simulink model "example_roboracer"  (R2024b)
settings: Solver=VariableStepAuto  StartTime=0.0  StopTime=inf  RelTol=1e-3
undefined symbols (not defined in the file or in its folder): gray
settings Model: Creator=tsamak  LastModifiedBy=tsamak
settings OptimizationCC: ZeroExternalMemoryAtStartup=off  ZeroInternalMemoryAtStartup=off  InitFltsAndDblsToZero=on
settings DebuggingCC: UnderSpecifiedDimensionMsg=warning
settings HardwareCC: ProdLongLongMode=on  TargetLongLongMode=on
settings SFSimCC: SimTargetLang=C++  GPUAcceleration=on  SimDLTargetLibrary=cudnn
settings RTWCC: TargetLang=C++  GenerateGPUCode=CUDA  GPUComputeCapability=3.5
settings GRTTargetCC: TargetLangStandard=C++11 (ISO)  CodeInterfacePackaging=C++ class

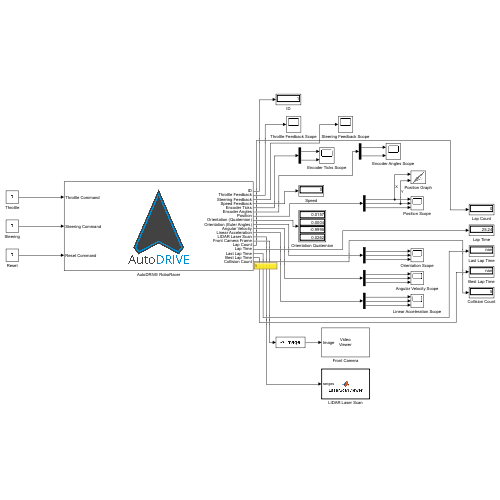
[thumbnail: Simulink's stored preview of the top-level diagram]
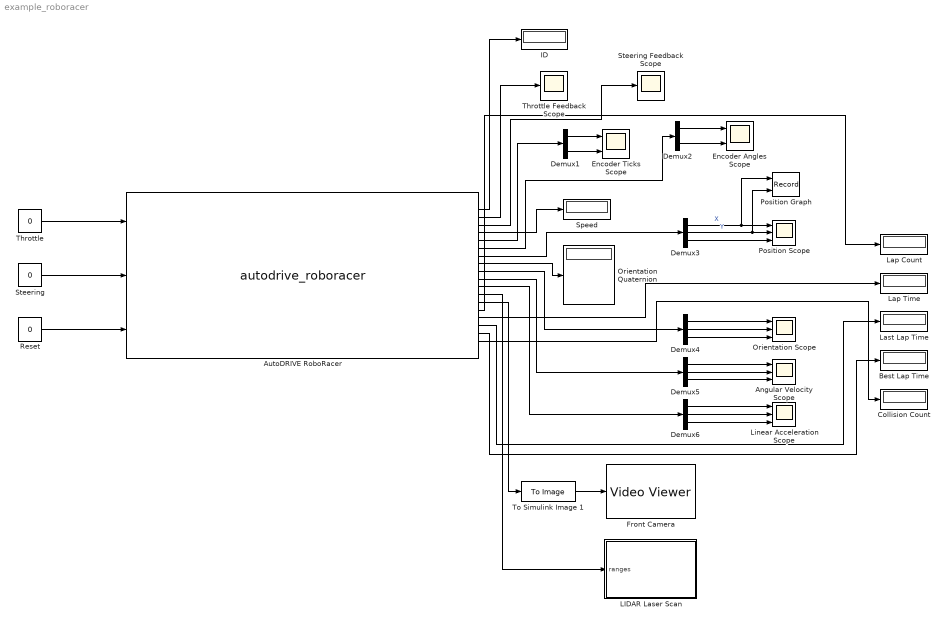
== system example_roboracer ==
  Angular Velocity Scope : Scope  NumInputPorts=3
  AutoDRIVE RoboRacer : M-S-Function  FunctionName=autodrive_roboracer  Parameters=Port  mask{Port=4567}
      mask Display:
      | image('autodrive_logo.png');
      | port_label('input', 1, 'Throttle Command');
      | port_label('input', 2, 'Steering Command');
      | port_label('input', 3, 'Reset Command');
      | port_label('output', 1, 'ID');
      | port_label('output', 2, 'Throttle Feedback');
      | port_label('output', 3, 'Steering Feedback');
      | port_label('output', 4, 'Speed Feedback');
      | port_label('output', 5, 'Encoder Ticks');
      | port_label('output', 6, 'Encoder Angles');
      | port_label('output', 7, 'Position');
      | port_label('output', 8, 'Orientation (Quaternion)');
      | port_label('output', 9, 'Orientation (Euler Angles)');
      | port_label('output', 10, 'Angular Velocity');
      | port_label('output', 11, 'Linear Acceleration');
      | port_label('output', 12, 'LIDAR Laser Scan');
      | port_label('output', 13, 'Front Camera Frame');
      | port_label('output', 14, 'Lap Count');
      | port_label('output', 15, 'Lap Time');
      | port_label('output', 16, 'Last Lap Time');
      | port_label('output', 17, 'Best Lap Time');
      | port_label('output', 18, 'Collision Count');
  Best Lap Time : Display
  Collision Count : Display
  Demux1 : Demux  Outputs=2
  Demux2 : Demux  Outputs=2
  Demux{3..6} (4 alike) : Demux  Outputs=3
  Encoder Angles Scope : Scope  NumInputPorts=2
  Encoder Ticks Scope : Scope  NumInputPorts=2
  Front Camera : VideoViewer  colormapValue=gray(256)  FigPos=[37 567.333333333333 408 304]
  ID : Display
  LIDAR Laser Scan : MATLAB Function  TreatAsAtomicUnit=on
  Lap Count : Display
  Lap Time : Display
  Last Lap Time : Display
  Linear Acceleration Scope : Scope  NumInputPorts=3
  Orientation Quaternion : Display
  Orientation Scope : Scope  NumInputPorts=3
  Position Graph : Record  FileSettingsInternal="{\"entries\":[{\"content\":{\"excelSettings\":{\"content\":{},\"type\":\"Streamout.ExcelSettings\"}},\"type\":\"Streamout.FileSettingStorage\",\"uuid\":\"\"}],\"packageUris\":[\"http:\\/\\/schema.mathworks.com\\/mf0\\/streamout_blocks\\/R2020a\"],\"version\":\"1.0\"}"  Layout=[1 1]  SignalsInternal="{\"entries\":[{\"content\":{\"signals\":[{\"content\":{\"blockPath\":[],\"dimensions\":[1,1],\"domain\":\"\",\"lineColor\":\"#139fff\",\"plots\":[ 1 ],\"port\":1,\"sid\":[\"\"],\"signalID\":1,\"signalName\":\"X\"},\"type\":\"RecordBlkView.Signal\",\"uuid\":\"\"},{\"content\":{\"blockPath\":[],\"dimensions\":[1,1],\"domain\":\"\",\"lineColor\":\"#139fff\",\"plots\":[ 1 ],\"port\":2,\"sid\":[\"\"],\"signalID\":2,\"signalName\":\"Y\"},\"type\":\"RecordBlkView.Signal\",\"uuid\":\"\"}]},\"type\":\"RecordBlkView.InputSignals\",\"uuid\":\"\"}],\"packageUris\":[\"http:\\/\\/schema.mathworks.com\\/mf0\\/streamout_blocks\\/R2020a\"],\"version\":\"1.0\"}"  VisualizationBindings="{\"xyplotplugin\":{\"info\":[{\"series\":[{\"bindingParametersList\":[{\"parameter\":\"X-Axis\",\"signalID\":1,\"signalName\":\"X\"},{\"parameter\":\"Y-Axis\",\"signalID\":2,\"signalName\":\"Y\"}],\"seriesID\":0}],\"subplotID\":1}]}}"  CompatibilityTag=XY
  Position Scope : Scope  NumInputPorts=3
  Reset : Constant  Value=0  OutDataTypeStr=uint16
  Speed : Display
  Steering : Constant  Value=0  OutDataTypeStr=double
  Steering Feedback Scope : Scope
  Throttle : Constant  Value=0  OutDataTypeStr=double
  Throttle Feedback Scope : Scope
  To Simulink Image 1 : ToImage
  wires:
  Demux3/2 -> Position Scope/2, Position Graph/2  "Y"
  Demux3/1 -> Position Scope/1, Position Graph/1  "X"
  Demux3/3 -> Position Scope/3
  AutoDRIVE RoboRacer/13 -> To Simulink Image 1/1
  To Simulink Image 1/1 -> Front Camera/1
  AutoDRIVE RoboRacer/7 -> Demux3/1
  AutoDRIVE RoboRacer/1 -> ID/1
  AutoDRIVE RoboRacer/2 -> Throttle Feedback Scope/1
  AutoDRIVE RoboRacer/3 -> Steering Feedback Scope/1
  AutoDRIVE RoboRacer/5 -> Demux1/1
  Demux1/1 -> Encoder Ticks Scope/1
  Demux1/2 -> Encoder Ticks Scope/2
  Demux2/1 -> Encoder Angles Scope/1
  Demux2/2 -> Encoder Angles Scope/2
  AutoDRIVE RoboRacer/6 -> Demux2/1
  Demux4/3 -> Orientation Scope/3
  Demux5/3 -> Angular Velocity Scope/3
  Demux6/3 -> Linear Acceleration Scope/3
  AutoDRIVE RoboRacer/8 -> Orientation Quaternion/1
  AutoDRIVE RoboRacer/9 -> Demux4/1
  AutoDRIVE RoboRacer/10 -> Demux5/1
  AutoDRIVE RoboRacer/11 -> Demux6/1
  Demux4/1 -> Orientation Scope/1
  Demux4/2 -> Orientation Scope/2
  Demux5/1 -> Angular Velocity Scope/1
  Demux5/2 -> Angular Velocity Scope/2
  Demux6/1 -> Linear Acceleration Scope/1
  Demux6/2 -> Linear Acceleration Scope/2
  Reset/1 -> AutoDRIVE RoboRacer/3
  Steering/1 -> AutoDRIVE RoboRacer/2
  Throttle/1 -> AutoDRIVE RoboRacer/1
  AutoDRIVE RoboRacer/4 -> Speed/1
  AutoDRIVE RoboRacer/14 -> Lap Count/1
  AutoDRIVE RoboRacer/15 -> Lap Time/1
  AutoDRIVE RoboRacer/16 -> Last Lap Time/1
  AutoDRIVE RoboRacer/17 -> Best Lap Time/1
  AutoDRIVE RoboRacer/18 -> Collision Count/1
  AutoDRIVE RoboRacer/12 -> LIDAR Laser Scan/1(ranges)

== matlab function example_roboracer/LIDAR Laser Scan ==
  data: ranges input
% function LaserScanViewer(ranges)
%     laserscan_fig = figure(1);
%     laserscan_ax = polaraxes;
%     angles = deg2rad(-45:0.25:225);
%     scatter(laserscan_ax, angles,ranges,1,'filled','red');
%     title('LIDAR Laser Scan');
%     drawnow;
% end

function LaserScanViewer(ranges)
    fig_tag = 'LaserScanViewerFig';
    fig_handle = findobj('Type', 'figure', 'Tag', fig_tag);

    if isempty(fig_handle)
        fig_handle = figure('Tag', fig_tag, 'Name', 'LIDAR', ...
                            'NumberTitle', 'off');
        polaraxes('Parent', fig_handle); % create axes inside figure
    end

    % Do not bring the figure to the foreground
    set(0, 'CurrentFigure', fig_handle);
    ax = findobj(fig_handle, 'Type', 'polaraxes');
    if isempty(ax)
        ax = polaraxes('Parent', fig_handle);
    end

    angles = deg2rad(-45:0.25:225);

    cla(ax);  % Clear previous plot
    scatter(ax, angles, ranges, 1, 'filled', 'red');
    title(ax, 'Laser Scan');

    drawnow limitrate;
end
